simulink model "stereoReverb"  (Simulink 7.7)
settings: Solver=FixedStepDiscrete  StartTime=0.0  StopTime=60  RelTol=1e-3
libraries: dspsigops x2, dspmtrx3 x2, dspsrcs4 x1, dspsnks4 x1
settings Model: Creator=Arun  LastModifiedBy=Arun

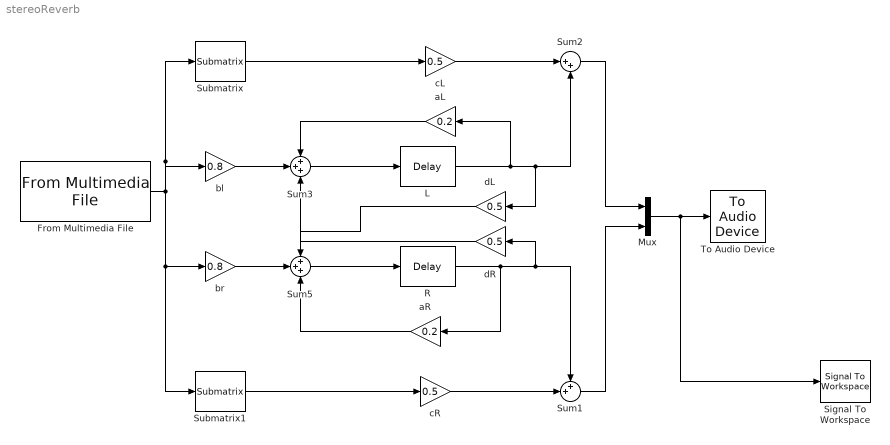
== system stereoReverb ==
  From Multimedia File : dspsrcs4/From Multimedia File  inputFilename=I:\Documents and Settings\Arun\My Documents\My Music\Vijay Yesudas, Swetha - www.123musiq.com - Casanovva\123 - Sakhiye - www.123musiq.com.WAV  loop=on  numPlays=1  outputStreams=Audio only  videoDataType=single  audioDataType=double  inheritSampleTime=on  userDefinedSampleTime=1/30  noAudioOutput=off  isIntensityVideo=off  fourcc=RGB  colorVideoFormat=Separate color signals  outputEOF=off  dataOrg=Column-major  audioFrameSize=1  computeAudioFrameSize=off
  L : dspsigops/Delay  InputProcessing=Columns as channels (frame based)  dly_unit=Samples  delay=3000  ic_detail=off  dif_ic_for_ch=off  dif_ic_for_dly=off  ic=0  reset_popup=None
  Mux : Mux  Inputs=2
  R : dspsigops/Delay  InputProcessing=Columns as channels (frame based)  dly_unit=Samples  delay=3000  ic_detail=off  dif_ic_for_ch=off  dif_ic_for_dly=off  ic=0  reset_popup=None
  Signal To Workspace : SignalToWorkspace  VariableName=audio_out  SaveFormat=Array  Save2DMode=2-D array (concatenate along first dimension)
      settings: CopyFcn=dspblkcopystw(gcbh);
  Submatrix : dspmtrx3/Submatrix  RowSpan=All rows  RowStartMode=First  RowStartIndex=1  RowEndMode=Last  RowEndIndex=1  ColSpan=One column  ColStartMode=First  ColStartIndex=1  ColEndMode=Last  ColEndIndex=1
  Submatrix1 : dspmtrx3/Submatrix  RowSpan=All rows  RowStartMode=First  RowStartIndex=1  RowEndMode=Last  RowEndIndex=1  ColSpan=One column  ColStartMode=Last  ColStartIndex=1  ColEndMode=Last  ColEndIndex=1
  Sum1 : Sum  Inputs=++|
  Sum2 : Sum  Inputs=|++
  Sum3 : Sum  Inputs=+++
  Sum5 : Sum  Inputs=+++
  To Audio Device : dspsnks4/To Audio Device  deviceName=Default  inheritSampleRate=on  sampleRate=44100  deviceDatatype=Determine from input data type  autoBufferSize=on  bufferSize=4096  queueDuration=1.0
  aL : Gain  Gain=0.2
  aR : Gain  Gain=0.2
  bl : Gain  Gain=0.8
  br : Gain  Gain=0.8
  cL : Gain  Gain=0.5
  cR : Gain  Gain=0.5
  dL : Gain  Gain=0.5
  dR : Gain  Gain=0.5
  wires:
  Submatrix/1 -> cL/1
  cL/1 -> Sum2/1
  L/1 -> aL/1, Sum2/2, dL/1
  aL/1 -> Sum3/1
  bl/1 -> Sum3/2
  Sum3/1 -> L/1
  From Multimedia File/1 -> Submatrix/1, bl/1, Submatrix1/1, br/1
  Submatrix1/1 -> cR/1
  R/1 -> aR/1, Sum1/1, dR/1
  Sum5/1 -> R/1
  aR/1 -> Sum5/3
  br/1 -> Sum5/2
  dR/1 -> Sum3/3
  dL/1 -> Sum5/1
  cR/1 -> Sum1/2
  Sum2/1 -> Mux/1
  Sum1/1 -> Mux/2
  Mux/1 -> To Audio Device/1, Signal To Workspace/1
